simulink model "Orbits"  (R2017a)
settings: Solver=VariableStepAuto  StartTime=0.0  StopTime=5*orb_time  FixedStep=24*60*60  MaxStep=orb_time*5e-3  MinStep=5e-2  RelTol=1e-6  EnableMultiTasking=on
model workspace (MATLAB code in the model file):
  | Orbits_Setup
undefined symbols (not defined in the file or in its folder): C1, C2, dec_year, Earth, EIRSAT1, k01, k02, k03, orb_time, WGS84, X, Y, Z
libraries: sm_lib x18, nesl_utility x12, cstblocks x6, sharedtransform x3, aerolibtransform2 x1, aerolibgravity2 x1
Description:
  | Copyright 2008-2016 The MathWorks, Inc.
settings Model: Creator=MathWorks  LastModifiedBy=vicctorio
settings SolverCC: ZeroCrossControl=EnableAll
settings DataIOCC: SaveFormat=Array  OutputTimes=0  ReturnWorkspaceOutputsName=out2
settings OptimizationCC: LifeSpan=inf
settings DebuggingCC: UnderspecifiedInitializationDetection=Classic  MergeDetectMultiDrivingBlocksExec=none  SolverPrmCheckMsg=warning  SFUnexpectedBacktrackingDiag=warning  SFNoUnconditionalDefaultTransitionDiag=warning  SFExecutionAtInitializationDiag=none
settings HardwareCC: ProdBitPerPointer=32  ProdBitPerSizeT=32  ProdBitPerPtrDiffT=32  ProdLargestAtomicFloat=None  ProdIntDivRoundTo=Undefined  ProdEndianess=Unspecified  ProdWordSize=32  ProdHWDeviceType=32-bit Generic
settings ModelReferenceCC: PropagateSignalLabelsOutOfModel=off
settings GRTTargetCC: TargetLangStandard=C89/C90 (ANSI)  GeneratePreprocessorConditionals=Disable all
settings ConfigComp: CovMetricSettings=dw  CovHtmlReporting=on  CovSaveCumulativeToWorkspaceVar=on  CovSaveSingleToWorkspaceVar=on  CovExternalEMLEnable=off
settings SimscapeCC: SimscapeLogLimitData=off
settings ConfigurationSet: Description=SimMechanics 2G
settings ExplorerConfigSet: InternalSimMechanicsExplorerSettings="<ExplorerConfiguration><canonicalview>default</canonicalview><AnimationSetting><BasePlaybackSpeed>1e3</BasePlaybackSpeed><PlaybackSpeedFactor>1.0</PlaybackSpeedFactor></AnimationSetting><TilePanel><TileInfo><Tiles Columns=\"2\" Count=\"4\" Rows=\"2\"><Column Left=\"2\" Weight=\"0.5\"/><Column Left=\"393\" Weight=\"0.5\"/><Column Left=\"784\"/><Row Top=\"2\" Weight=\"0.5\"/><Row Top=\"345\" Weight=\"0.5\"/><Row Top=\"688\"/><Tile Height=\"1\" Width=\"1\" X=\"0\" Y=\"0\"/><Tile Height=\"1\" Width=\"1\" X=\"0\" Y=\"1\"/><Tile Height=\"1\" Width=\"1\" X=\"1\" Y=\"0\"/><Tile Height=\"1\" Width=\"1\" X=\"1\" Y=\"1\"/></Tiles></TileInfo><SceneInfo><SceneViewer><BGColor><R>0.901960790157318115</R><G>0.901960790157318115</G><B>0.901960790157318115</B></BGColor><Camera><DoPerspective>off</DoPerspective><Position><X>-203.545490264892578</X><Y>-167484806.482812434</Y><Z>-58.7216796875145519</Z></Position><Center><X>-203.545490264892578</X><Y>-83700.054443359375</Y><Z>-58.7216796875145519</Z></Center><Up><X>0</X><Y>-0</Y><Z>1</Z></Up><ViewLimDist>1</ViewLimDist><YLim>6562130</YLim><XLim>7505190.59880239516</XLim></Camera></SceneViewer><SceneViewer><BGColor><R>0.901960790157318115</R><G>0.901960790157318115</G><B>0.901960790157318115</B></BGColor><Camera><DoPerspective>off</DoPerspective><Position><X>-99808.0000004172325</X><Y>1.9073486328125e-06</Y><Z>11080569.0027875006</Z></Position><Center><X>-99808.0000004172325</X><Y>1.9073486328125e-06</Y><Z>1541215.53125</Z></Center><Up><X>0</X><Y>1</Y><Z>-0</Z></Up><ViewLimDist>1</ViewLimDist><YLim>7206500.06000000052</YLim><XLim>8242164.73928143829</XLim></Camera></SceneViewer><SceneViewer><BGColor><R>0.901960790157318115</R><G>0.901960790157318115</G><B>0.901960790157318115</B></BGColor><Camera><DoPerspective>off</DoPerspective><Position><X>1780793989.13458633</X><Y>-0.765625</Y><Z>0.0923618078231811523</Z></Position><Center><X>-1228213.1171875</X><Y>-0.765625</Y><Z>0.0923618078231811523</Z></Center><Up><X>-0</X><Y>0</Y><Z>1</Z></Up><ViewLimDist>1</ViewLimDist><YLim>6860208.48896073923</YLim><XLim>7846106.71491916943</XLim></Camera></SceneViewer><SceneViewer><BGColor><R>0.901960790157318115</R><G>0.901960790157318115</G><B>0.901960790157318115</B></BGColor><Camera><DoPerspective>off</DoPerspective><Position><X>1473413538.72739792</X><Y>-1473413538.82131076</Y><Z>1473411667.66141582</Z></Position><Center><X>-14.9597511113855024</X><Y>14.8658383234217677</Y><Z>-15.3674730430210413</Z></Center><Up><X>-0.408248290463863073</X><Y>0.408248290463863073</Y><Z>0.816496580927726145</Z></Up><ViewLimDist>1</ViewLimDist><YLim>10412227.7699999996</YLim><XLim>11908595.8327544909</XLim></Camera></SceneViewer></SceneInfo></TilePanel><MechEditorPanel><Cameras/><GfxPanelCameraMap/></MechEditorPanel></ExplorerConfiguration>"

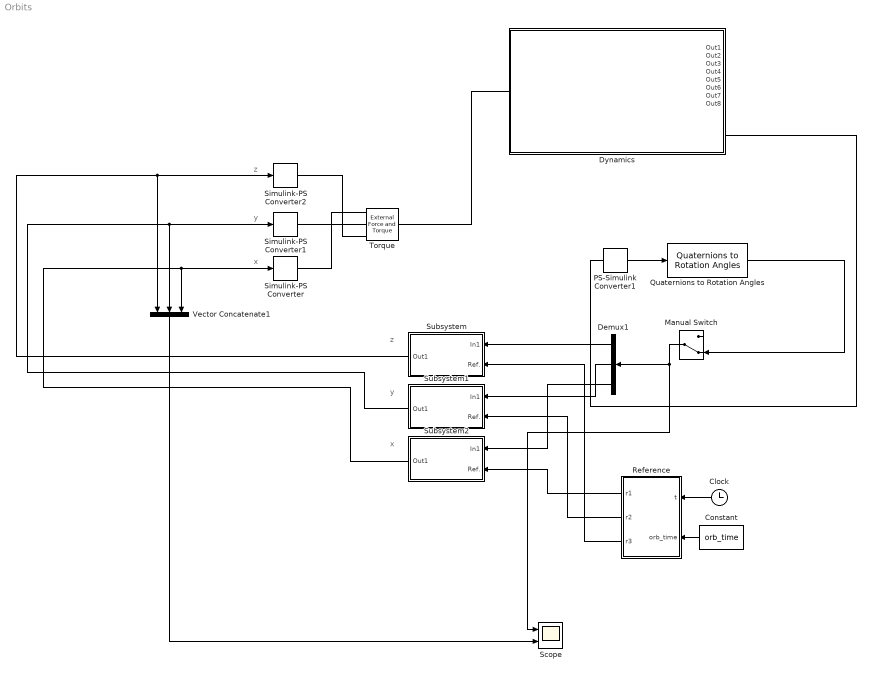
== system Orbits ==
  note: x
  note: y
  note: z
  note: x
  note: y
  note: z
  Clock : Clock
  Constant : Constant  Value=orb_time
  Demux1 : Demux  Outputs=3
  Dynamics : Subsystem
  Manual Switch : ManualSwitch  CurrentSetting=0
  PS-Simulink Converter1 : nesl_utility/PS-Simulink Converter  PhysicalDomain=network_engine_domain  SubClassName=ps_output  LeftPortType=input  RightPortType=output  PseudoPeriodic=off  Frequencies=[]  Unit=1  AffineConversion=off
  Quaternions to Rotation Angles : sharedtransform/Quaternions to Rotation Angles  rotationOrder=ZYX
  Reference : MATLAB Function  TreatAsAtomicUnit=on
  Scope : Scope  NumInputPorts=2
  Simulink-PS Converter : nesl_utility/Simulink-PS Converter  PhysicalDomain=network_engine_domain  SubClassName=ps_input  LeftPortType=input  RightPortType=output  PseudoPeriodic=off  Frequencies=[]  NoiseDistribution=none  NoiseParameters=[]  Unit=1  AffineConversion=off  FilteringAndDerivatives=zero  SimscapeFilterOrder=1  InputFilterTimeConstant=0.001  UdotUserProvided=1
  Simulink-PS Converter1 : nesl_utility/Simulink-PS Converter  PhysicalDomain=network_engine_domain  SubClassName=ps_input  LeftPortType=input  RightPortType=output  PseudoPeriodic=off  Frequencies=[]  NoiseDistribution=none  NoiseParameters=[]  Unit=1  AffineConversion=off  FilteringAndDerivatives=zero  SimscapeFilterOrder=1  InputFilterTimeConstant=0.001  UdotUserProvided=1
  Simulink-PS Converter2 : nesl_utility/Simulink-PS Converter  PhysicalDomain=network_engine_domain  SubClassName=ps_input  LeftPortType=input  RightPortType=output  PseudoPeriodic=off  Frequencies=[]  NoiseDistribution=none  NoiseParameters=[]  Unit=1  AffineConversion=off  FilteringAndDerivatives=zero  SimscapeFilterOrder=1  InputFilterTimeConstant=0.001  UdotUserProvided=1
  Subsystem : Subsystem
  Subsystem1 : Subsystem
  Subsystem2 : Subsystem
  Torque : sm_lib/Forces and Torques/External Force and Torque  ForceResolutionFrame=AttachedFrame  EnableForceX=off  EnableForceY=off  EnableForceZ=off  EnableForce=off  TorqueResolutionFrame=AttachedFrame  EnableTorqueX=on  EnableTorqueY=on  EnableTorqueZ=on  EnableTorque=off
  Vector Concatenate1 : Concatenate  NumInputs=3
  wires:
  PS-Simulink Converter1/1 -> Quaternions to Rotation Angles/1
  Demux1/2 -> Subsystem1/1(In1)
  Demux1/1 -> Subsystem/1(In1)
  Demux1/3 -> Subsystem2/1(In1)
  Quaternions to Rotation Angles/1 -> Manual Switch/2
  Vector Concatenate1/1 -> Scope/2
  Manual Switch/1 -> Scope/1, Demux1/1
  Clock/1 -> Reference/1(t)
  Constant/1 -> Reference/2(orb_time)
  Reference/2(r2) -> Subsystem1/2(Ref.)
  Reference/1(r1) -> Subsystem2/2(Ref.)
  Reference/3(r3) -> Subsystem/2(Ref.)
  Subsystem/1(Out1) -> Simulink-PS Converter2/1, Vector Concatenate1/1
  Subsystem1/1(Out1) -> Simulink-PS Converter1/1, Vector Concatenate1/2
  Subsystem2/1(Out1) -> Simulink-PS Converter/1, Vector Concatenate1/3
  connections:
  Simulink-PS Converter1/RConn1 -- Torque/LConn2
  Simulink-PS Converter/RConn1 -- Torque/LConn1
  Simulink-PS Converter2/RConn1 -- Torque/LConn3
  Torque/RConn1 -- Dynamics/LConn1
  Dynamics/RConn4 -- PS-Simulink Converter1/LConn1

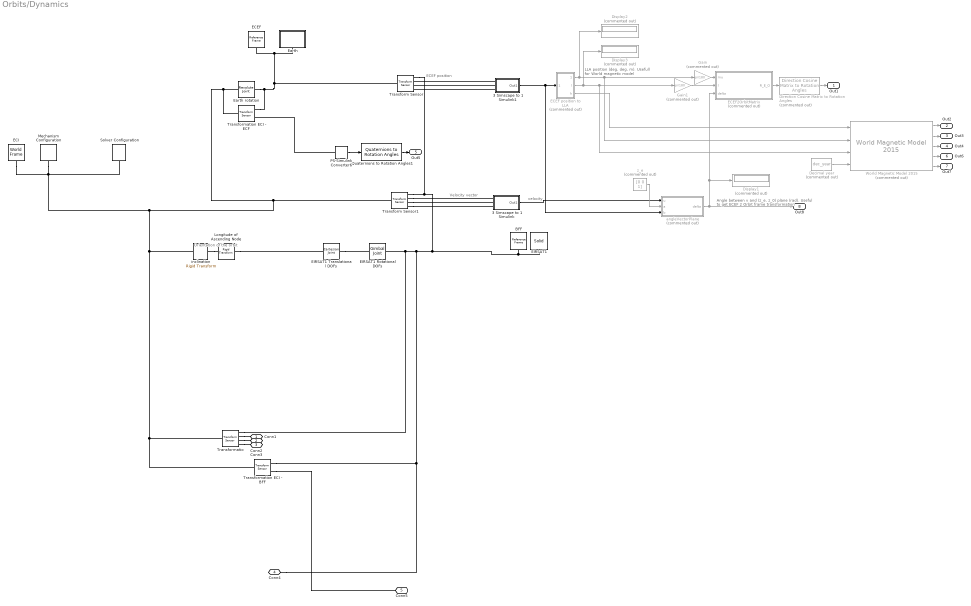
== system Orbits/Dynamics ==
  note: LLA position (deg, deg, m).
      | Usefull for World magnetic model
  note: Angle between v and (z_e, z_0) plane (rad).
      | Useful to get ECEF 2 Orbit frame transformation
  note: velocity
  note: Velocity vector
  note: ECEF position
  note: Orientation of the orbit
  " Earth rotation" : sm_lib/Joints/Revolute Joint  SenseConstraintForce=off  SenseConstraintForceX=off  SenseConstraintForceY=off  SenseConstraintForceZ=off  SenseConstraintTorque=off  SenseConstraintTorqueX=off  SenseConstraintTorqueY=off  SenseConstraintTorqueZ=off  SenseTotalForce=off  SenseTotalForceX=off  SenseTotalForceY=off  SenseTotalForceZ=off  SenseTotalTorque=off  SenseTotalTorqueX=off  SenseTotalTorqueY=off  SenseTotalTorqueZ=off  CompositeWrenchDir=FollowerOnBase  CompositeWrenchFrame=BaseFrame  EquilibriumPosition=0  EquilibriumPositionUnits=deg  SpringStiffness=0  SpringStiffnessUnits=N*m/deg  DampingCoefficient=0  DampingCoefficientUnits=N*m/(deg/s)  TorqueActuationMode=NoTorque  MotionActuationMode=ComputedMotion  SensePosition=off  SenseVelocity=off  SenseAcceleration=off  SenseTorqueForce=off  PositionTargetSpecify=off  PositionTargetPriority=High  PositionTargetValue=0  PositionTargetValueUnits=deg  VelocityTargetSpecify=on  VelocityTargetPriority=High  VelocityTargetValue=Earth.w  VelocityTargetValueUnits=deg/s
  3 Simscape to 1 Simulink : Subsystem
  3 Simscape to 1 Simulink1 : Subsystem
  BFF : sm_lib/Frames and Transforms/Reference Frame
  Decimal year : Constant  Commented=on  Value=dec_year
  Direction Cosine Matrix to Rotation Angles : sharedtransform/Direction Cosine Matrix to Rotation Angles  Commented=on  rotationOrder=ZYX  lim=Default
  Display1 : Display  Commented=on
  Display2 : Display  Commented=on
  Display3 : Display  Commented=on
  "ECEF " : sm_lib/Frames and Transforms/Reference Frame
  ECEF position to LLA : Subsystem  Commented=on
  ECEF2OrbitMatrix : MATLAB Function  Commented=on  TreatAsAtomicUnit=on
  ECI : sm_lib/Frames and Transforms/World Frame
  EIRSAT1 : sm_lib/Body Elements/Solid  InertiaType=Custom  Mass=EIRSAT1.M  MassUnits=kg  CenterOfMass=EIRSAT1.COM  CenterOfMassUnits=m  MomentsOfInertia=EIRSAT1.MomI  MomentsOfInertiaUnits=kg*m^2  ProductsOfInertia=EIRSAT1.ProdI  ProductsOfInertiaUnits=kg*m^2  DensityBased=off  Density=1000  DensityUnits=kg/(m^3)  DoExposeReferenceFrame=on  SerializedFrames=<Frames/>  GraphicType=FromGeometry  MarkerShape=Sphere  MarkerSize=10  MarkerSizeUnits=m  GraphicVisPropType=SimpleVisualProperties  GraphicDiffuseColor=EIRSAT1.RGB  GraphicSpecularColor=[0.5 0.5 0.5 1.0]  GraphicAmbientColor=[0.15 0.15 0.15 1.0]  GraphicEmissiveColor=[0.0 0.0 0.0 1.0]  GraphicShininess=75  GraphicOpacity=1.0  GeometryShape=Brick  RectangleSize=[1 1]  RectangleSizeUnits=m  BrickDimensions=[1 1 2] * EIRSAT1.R  BrickDimensionUnits=m  CylinderRadius=1  CylinderRadiusUnits=m  CylinderLength=1  CylinderLengthUnits=m  SphereRadius=EIRSAT1.R  SphereRadiusUnits=m  EllipsoidRadii=[1 1 1]  EllipsoidRadiiUnits=m  ExtrusionCrossSection=[1 1; -1 1; -1 -1; 1 -1]  ExtrusionCrossSectionUnits=m  ExtrusionLength=1  ExtrusionLengthUnits=m  PolygonNumSides=3  PolygonOuterRadius=1  PolygonOuterRadiusUnits=m  ExtGeomFileType=STL  ExtGeomFileUnits=m  RevolutionCrossSection=[1 1; 1 -1; 2 -1; 2 1]  RevolutionCrossSectionUnits=m  RevolutionExtent=Full  RevolutionAngle=180  RevolutionAngleUnits=deg
  EIRSAT1 Rotational DOFs : sm_lib/Joints/Gimbal Joint  SenseConstraintForce=off  SenseConstraintForceX=off  SenseConstraintForceY=off  SenseConstraintForceZ=off  SenseConstraintTorque=off  SenseConstraintTorqueX=off  SenseConstraintTorqueY=off  SenseConstraintTorqueZ=off  SenseTotalForce=off  SenseTotalForceX=off  SenseTotalForceY=off  SenseTotalForceZ=off  SenseTotalTorque=off  SenseTotalTorqueX=off  SenseTotalTorqueY=off  SenseTotalTorqueZ=off  CompositeWrenchDir=FollowerOnBase  CompositeWrenchFrame=BaseFrame  RxEquilibriumPosition=0  RxEquilibriumPositionUnits=deg  RxSpringStiffness=0  RxSpringStiffnessUnits=N*m/deg  RxDampingCoefficient=0  RxDampingCoefficientUnits=N*m/(deg/s)  RxTorqueActuationMode=NoTorque  RxMotionActuationMode=ComputedMotion  RxSensePosition=off  RxSenseVelocity=off  RxSenseAcceleration=off  RxSenseTorqueForce=off  RxPositionTargetSpecify=off  RxPositionTargetPriority=High  RxPositionTargetValue=0  RxPositionTargetValueUnits=deg  RxVelocityTargetSpecify=off  RxVelocityTargetPriority=High  RxVelocityTargetValue=0.2  RxVelocityTargetValueUnits=rad/s  RyEquilibriumPosition=0  RyEquilibriumPositionUnits=deg  RySpringStiffness=0  RySpringStiffnessUnits=N*m/deg  RyDampingCoefficient=0  RyDampingCoefficientUnits=N*m/(deg/s)  RyTorqueActuationMode=NoTorque  RyMotionActuationMode=ComputedMotion  RySensePosition=off  RySenseVelocity=off  RySenseAcceleration=off  RySenseTorqueForce=off  RyPositionTargetSpecify=off  RyPositionTargetPriority=High  RyPositionTargetValue=0  RyPositionTargetValueUnits=deg  RyVelocityTargetSpecify=off  RyVelocityTargetPriority=High  RyVelocityTargetValue=0.1  RyVelocityTargetValueUnits=deg/s  RzEquilibriumPosition=0  RzEquilibriumPositionUnits=deg  RzSpringStiffness=0  RzSpringStiffnessUnits=N*m/deg  RzDampingCoefficient=0  RzDampingCoefficientUnits=N*m/(deg/s)  RzTorqueActuationMode=NoTorque  RzMotionActuationMode=ComputedMotion  RzSensePosition=off  RzSenseVelocity=off  RzSenseAcceleration=off  RzSenseTorqueForce=off  RzPositionTargetSpecify=off  RzPositionTargetPriority=High  RzPositionTargetValue=0  RzPositionTargetValueUnits=deg  RzVelocityTargetSpecify=off  RzVelocityTargetPriority=High  RzVelocityTargetValue=0.1  RzVelocityTargetValueUnits=deg/s
      settings: SourceProductName=Simscape Multibody
  EIRSAT1 Translational DOFs : sm_lib/Joints/Cartesian Joint  SenseConstraintForce=off  SenseConstraintForceX=off  SenseConstraintForceY=off  SenseConstraintForceZ=off  SenseConstraintTorque=off  SenseConstraintTorqueX=off  SenseConstraintTorqueY=off  SenseConstraintTorqueZ=off  SenseTotalForce=off  SenseTotalForceX=off  SenseTotalForceY=off  SenseTotalForceZ=off  SenseTotalTorque=off  SenseTotalTorqueX=off  SenseTotalTorqueY=off  SenseTotalTorqueZ=off  CompositeWrenchDir=FollowerOnBase  CompositeWrenchFrame=BaseFrame  PxEquilibriumPosition=0  PxEquilibriumPositionUnits=m  PxSpringStiffness=0  PxSpringStiffnessUnits=N/m  PxDampingCoefficient=0  PxDampingCoefficientUnits=N/(m/s)  PxTorqueActuationMode=NoTorque  PxMotionActuationMode=ComputedMotion  PxSensePosition=off  PxSenseVelocity=off  PxSenseAcceleration=off  PxSenseTorqueForce=off  PxPositionTargetSpecify=on  PxPositionTargetPriority=High  PxPositionTargetValue=EIRSAT1.Px  PxPositionTargetValueUnits=m  PxVelocityTargetSpecify=on  PxVelocityTargetPriority=High  PxVelocityTargetValue=EIRSAT1.Vx  PxVelocityTargetValueUnits=m/s  PyEquilibriumPosition=0  PyEquilibriumPositionUnits=m  PySpringStiffness=0  PySpringStiffnessUnits=N/m  PyDampingCoefficient=0  PyDampingCoefficientUnits=N/(m/s)  PyTorqueActuationMode=NoTorque  PyMotionActuationMode=ComputedMotion  PySensePosition=off  PySenseVelocity=off  PySenseAcceleration=off  PySenseTorqueForce=off  PyPositionTargetSpecify=on  PyPositionTargetPriority=High  PyPositionTargetValue=EIRSAT1.Py  PyPositionTargetValueUnits=m  PyVelocityTargetSpecify=on  PyVelocityTargetPriority=High  PyVelocityTargetValue=EIRSAT1.Vy  PyVelocityTargetValueUnits=m/s  PzEquilibriumPosition=0  PzEquilibriumPositionUnits=m  PzSpringStiffness=0  PzSpringStiffnessUnits=N/m  PzDampingCoefficient=0  PzDampingCoefficientUnits=N/(m/s)  PzTorqueActuationMode=NoTorque  PzMotionActuationMode=ComputedMotion  PzSensePosition=off  PzSenseVelocity=off  PzSenseAcceleration=off  PzSenseTorqueForce=off  PzPositionTargetSpecify=off  PzPositionTargetPriority=High  PzPositionTargetValue=0  PzPositionTargetValueUnits=m  PzVelocityTargetSpecify=off  PzVelocityTargetPriority=High  PzVelocityTargetValue=0  PzVelocityTargetValueUnits=m/s
  Earth : Subsystem
  Gain : Gain  Commented=on  Gain=pi/180
  Gain1 : Gain  Commented=on  Gain=pi/180
  Longitude of Ascending Node : sm_lib/Frames and Transforms/Rigid Transform  TranslationMethod=None  TranslationStandardOffset=0  TranslationLengthUnit=m  TranslationStandardAxis=+Z  TranslationCartesianOffset=[0 0 0]  TranslationROffset=0  TranslationROffsetUnits=m  TranslationZOffset=0  TranslationZOffsetUnits=m  TranslationThetaOffset=0  TranslationThetaOffsetUnits=deg  RotationMethod=StandardAxis  RotationAngleUnits=deg  RotationStandardAxis=+Z  RotationAngle=48.33  RotationArbitraryAxis=[0 0 1]  FollAlignAxisA=+X  BaseAlignAxisA=+Y  FollAlignAxisB=+Y  BaseAlignAxisB=+Z  RotationSequenceAxes=FollowerAxes  RotationSequence=XYX  RotationSequenceAngles=[0 0 0]  RotationSequenceAnglesUnits=deg  RotationMatrix=[1 0 0; 0 1 0; 0 0 1]
  Mechanism Configuration : sm_lib/Utilities/Mechanism Configuration  UniformGravity=None  GravityVector=[0 0 -9.80665]  GravityUnits=m/s^2  LinearizationDelta=0.001
  PS-Simulink Converter6 : nesl_utility/PS-Simulink Converter  PhysicalDomain=network_engine_domain  SubClassName=ps_output  LeftPortType=input  RightPortType=output  PseudoPeriodic=off  Frequencies=[]  Unit=1  AffineConversion=off
  Quaternions to Rotation Angles1 : sharedtransform/Quaternions to Rotation Angles  rotationOrder=ZYX
  Solver Configuration : nesl_utility/Solver Configuration  PhysicalDomain=network_engine_domain  SubClassName=solver  LeftPortType=input  RightPortType=generic  Accelerate=off  Tones=[]  Harmonics=[]  SimulateNoise=off  Profile=off  UseLocalSampling=off  EnableSwitchedLinearOptims=on  FrequencyDomain=off  UseCCode=off  RelTol=0.001  AbsTol=1e-06  MinStep=1e-09  ToWorkspace=off  RevertToSquareIcSolve=off  NumHomotopyIterations=100  PhasorMode=off  PhasorModeNumHarmonics=1  OverrideAbsTol=off  DoDC=off  ResidualTolerance=1e-09  UseLocalSolver=off  LocalSolverChoice=NE_BACKWARD_EULER_ADVANCER  LocalSolverSampleTime=0.001  DoFixedCost=off  MaxNonlinIter=3  MaxModeIter=2  LinearAlgebra=Sparse  DelaysMemoryBudget=1024  AutomaticFiltering=on  FilteringTimeConstant=0.001
  Transform Sensor : sm_lib/Frames and Transforms/Transform Sensor  MeasurementFrame=World  SenseAngle=off  SenseAxis=off  SenseAngle1=off  SenseAngle2=off  SenseAngle3=off  SenseQ=off  SenseR=off  SenseOmegaX=off  SenseOmegaY=off  SenseOmegaZ=off  SenseOmega1=off  SenseOmega2=off  SenseOmega3=off  SenseQDot=off  SenseRDot=off  SenseAlphaX=off  SenseAlphaY=off  SenseAlphaZ=off  SenseAlpha1=off  SenseAlpha2=off  SenseAlpha3=off  SenseQDDot=off  SenseRDDot=off  SenseX=on  SenseY=on  SenseZ=on  SenseRad=off  SenseAzim=off  SenseDist=off  SenseInc=off  SenseXDot=off  SenseYDot=off  SenseZDot=off  SenseRadDot=off  SenseAzimDot=off  SenseDistDot=off  SenseIncDot=off  SenseXDDot=off  SenseYDDot=off  SenseZDDot=off  SenseRadDDot=off  SenseAzimDDot=off  SenseDistDDot=off  SenseIncDDot=off
  Transform Sensor1 : sm_lib/Frames and Transforms/Transform Sensor  MeasurementFrame=World  SenseAngle=off  SenseAxis=off  SenseAngle1=off  SenseAngle2=off  SenseAngle3=off  SenseQ=off  SenseR=off  SenseOmegaX=off  SenseOmegaY=off  SenseOmegaZ=off  SenseOmega1=off  SenseOmega2=off  SenseOmega3=off  SenseQDot=off  SenseRDot=off  SenseAlphaX=off  SenseAlphaY=off  SenseAlphaZ=off  SenseAlpha1=off  SenseAlpha2=off  SenseAlpha3=off  SenseQDDot=off  SenseRDDot=off  SenseX=off  SenseY=off  SenseZ=off  SenseRad=off  SenseAzim=off  SenseDist=off  SenseInc=off  SenseXDot=on  SenseYDot=on  SenseZDot=on  SenseRadDot=off  SenseAzimDot=off  SenseDistDot=off  SenseIncDot=off  SenseXDDot=off  SenseYDDot=off  SenseZDDot=off  SenseRadDDot=off  SenseAzimDDot=off  SenseDistDDot=off  SenseIncDDot=off
  Transformatio : sm_lib/Frames and Transforms/Transform Sensor  MeasurementFrame=World  SenseAngle=off  SenseAxis=off  SenseAngle1=off  SenseAngle2=off  SenseAngle3=off  SenseQ=off  SenseR=off  SenseOmegaX=off  SenseOmegaY=off  SenseOmegaZ=off  SenseOmega1=off  SenseOmega2=off  SenseOmega3=off  SenseQDot=off  SenseRDot=off  SenseAlphaX=off  SenseAlphaY=off  SenseAlphaZ=off  SenseAlpha1=off  SenseAlpha2=off  SenseAlpha3=off  SenseQDDot=off  SenseRDDot=off  SenseX=on  SenseY=on  SenseZ=on  SenseRad=off  SenseAzim=off  SenseDist=off  SenseInc=off  SenseXDot=off  SenseYDot=off  SenseZDot=off  SenseRadDot=off  SenseAzimDot=off  SenseDistDot=off  SenseIncDot=off  SenseXDDot=off  SenseYDDot=off  SenseZDDot=off  SenseRadDDot=off  SenseAzimDDot=off  SenseDistDDot=off  SenseIncDDot=off
  Transformation ECI - BFF : sm_lib/Frames and Transforms/Transform Sensor  MeasurementFrame=World  SenseAngle=off  SenseAxis=off  SenseAngle1=off  SenseAngle2=off  SenseAngle3=off  SenseQ=on  SenseR=off  SenseOmegaX=off  SenseOmegaY=off  SenseOmegaZ=off  SenseOmega1=off  SenseOmega2=off  SenseOmega3=off  SenseQDot=off  SenseRDot=off  SenseAlphaX=off  SenseAlphaY=off  SenseAlphaZ=off  SenseAlpha1=off  SenseAlpha2=off  SenseAlpha3=off  SenseQDDot=off  SenseRDDot=off  SenseX=off  SenseY=off  SenseZ=off  SenseRad=off  SenseAzim=off  SenseDist=off  SenseInc=off  SenseXDot=off  SenseYDot=off  SenseZDot=off  SenseRadDot=off  SenseAzimDot=off  SenseDistDot=off  SenseIncDot=off  SenseXDDot=off  SenseYDDot=off  SenseZDDot=off  SenseRadDDot=off  SenseAzimDDot=off  SenseDistDDot=off  SenseIncDDot=off
  Transformation ECI - ECF : sm_lib/Frames and Transforms/Transform Sensor  MeasurementFrame=World  SenseAngle=off  SenseAxis=off  SenseAngle1=off  SenseAngle2=off  SenseAngle3=off  SenseQ=on  SenseR=off  SenseOmegaX=off  SenseOmegaY=off  SenseOmegaZ=off  SenseOmega1=off  SenseOmega2=off  SenseOmega3=off  SenseQDot=off  SenseRDot=off  SenseAlphaX=off  SenseAlphaY=off  SenseAlphaZ=off  SenseAlpha1=off  SenseAlpha2=off  SenseAlpha3=off  SenseQDDot=off  SenseRDDot=off  SenseX=off  SenseY=off  SenseZ=off  SenseRad=off  SenseAzim=off  SenseDist=off  SenseInc=off  SenseXDot=off  SenseYDot=off  SenseZDot=off  SenseRadDot=off  SenseAzimDot=off  SenseDistDot=off  SenseIncDot=off  SenseXDDot=off  SenseYDDot=off  SenseZDDot=off  SenseRadDDot=off  SenseAzimDDot=off  SenseDistDDot=off  SenseIncDDot=off
  World Magnetic Model 2015 : aerolibgravity2/World Magnetic Model 2015  Commented=on  units=Metric (MKS)  time_in=on  month=January  day=1  year=2015  action=Error  h_out=on  dec_out=on  inc_out=on  ti_out=on
      settings: SourceProductName=Aerospace Blockset  SourceProductBaseCode=AE
  angleVectorPlane : MATLAB Function  Commented=on  TreatAsAtomicUnit=on
  inclination : sm_lib/Frames and Transforms/Rigid Transform  TranslationMethod=None  TranslationStandardOffset=0  TranslationLengthUnit=m  TranslationStandardAxis=+Z  TranslationCartesianOffset=[0 0 0]  TranslationROffset=0  TranslationROffsetUnits=m  TranslationZOffset=0  TranslationZOffsetUnits=m  TranslationThetaOffset=0  TranslationThetaOffsetUnits=deg  RotationMethod=StandardAxis  RotationAngleUnits=deg  RotationStandardAxis=+X  RotationAngle=20  RotationArbitraryAxis=[0 0 1]  FollAlignAxisA=+X  BaseAlignAxisA=+Y  FollAlignAxisB=+Y  BaseAlignAxisB=+Z  RotationSequenceAxes=FollowerAxes  RotationSequence=XYX  RotationSequenceAngles=[0 0 0]  RotationSequenceAnglesUnits=deg  RotationMatrix=[1 0 0; 0 1 0; 0 0 1]
  z_e : Constant  Commented=on  Value=[0 0 1]
  Conn1 : PMIOPort  Port=1  Side=Right
  Conn2 : PMIOPort  Port=2  Side=Right
  Conn3 : PMIOPort  Port=3  Side=Right
  Conn4 : PMIOPort  Port=4  Side=Left
  Conn5 : PMIOPort  Port=5  Side=Right
  Out1 : Outport
  Out2 : Outport  Port=2
  Out3 : Outport  Port=3
  Out4 : Outport  Port=4
  Out5 : Outport  Port=5
  Out6 : Outport  Port=6
  Out7 : Outport  Port=7
  Out8 : Outport  Port=8
  wires:
  PS-Simulink Converter6/1 -> Quaternions to Rotation Angles1/1
  3 Simscape to 1 Simulink/1(Out1) -> angleVectorPlane/1(u)
  ECEF position to LLA/2(l) -> Display3/1, World Magnetic Model 2015/3, Gain1/1
  3 Simscape to 1 Simulink1/1(Out1) -> angleVectorPlane/3(b), ECEF position to LLA/1(In1)
  Gain1/1 -> ECEF2OrbitMatrix/2(l)
  z_e/1 -> angleVectorPlane/2(a)
  angleVectorPlane/1(delta) -> Out8/1, ECEF2OrbitMatrix/3(delta), Display1/1
  Decimal year/1 -> World Magnetic Model 2015/4
  ECEF position to LLA/3(h) -> World Magnetic Model 2015/1
  ECEF2OrbitMatrix/1(R_E_O) -> Direction Cosine Matrix to Rotation Angles/1
  ECEF position to LLA/1(mu) -> Gain/1, World Magnetic Model 2015/2, Display2/1
  Gain/1 -> ECEF2OrbitMatrix/1(mu)
  World Magnetic Model 2015/3 -> Out4/1
  Quaternions to Rotation Angles1/1 -> Out5/1
  World Magnetic Model 2015/1 -> Out2/1
  World Magnetic Model 2015/4 -> Out6/1
  World Magnetic Model 2015/5 -> Out7/1
  Direction Cosine Matrix to Rotation Angles/1 -> Out1/1
  World Magnetic Model 2015/2 -> Out3/1
  connections:
  Transformation ECI - BFF/RConn2 -- Conn5/RConn1
  inclination/RConn1 -- Longitude of Ascending Node/LConn1
  inclination/LConn1 -- Transformatio/LConn1 -- Transformation ECI - BFF/LConn1 -- " Earth rotation"/LConn1 -- Transformation ECI - ECF/LConn1 -- Transform Sensor1/LConn1 -- Solver Configuration/RConn1 -- ECI/RConn1 -- Mechanism Configuration/RConn1
  Transformation ECI - BFF/RConn1 -- Conn4/RConn1 -- EIRSAT1/RConn1 -- BFF/RConn1 -- Transform Sensor/RConn1 -- Transform Sensor1/RConn1 -- Transformatio/RConn1 -- EIRSAT1 Rotational DOFs/RConn1
  Longitude of Ascending Node/RConn1 -- EIRSAT1 Translational DOFs/LConn1
  PS-Simulink Converter6/LConn1 -- Transformation ECI - ECF/RConn2
  " Earth rotation"/RConn1 -- Transform Sensor/LConn1 -- Earth/LConn1 -- "ECEF "/RConn1 -- Transformation ECI - ECF/RConn1
  Transform Sensor1/RConn4 -- 3 Simscape to 1 Simulink/LConn3
  Transform Sensor1/RConn2 -- 3 Simscape to 1 Simulink/LConn1
  EIRSAT1 Translational DOFs/RConn1 -- EIRSAT1 Rotational DOFs/LConn1
  Transform Sensor1/RConn3 -- 3 Simscape to 1 Simulink/LConn2
  3 Simscape to 1 Simulink1/LConn3 -- Transform Sensor/RConn4
  3 Simscape to 1 Simulink1/LConn1 -- Transform Sensor/RConn2
  3 Simscape to 1 Simulink1/LConn2 -- Transform Sensor/RConn3
  Transformatio/RConn2 -- Conn1/RConn1
  Transformatio/RConn3 -- Conn2/RConn1
  Transformatio/RConn4 -- Conn3/RConn1

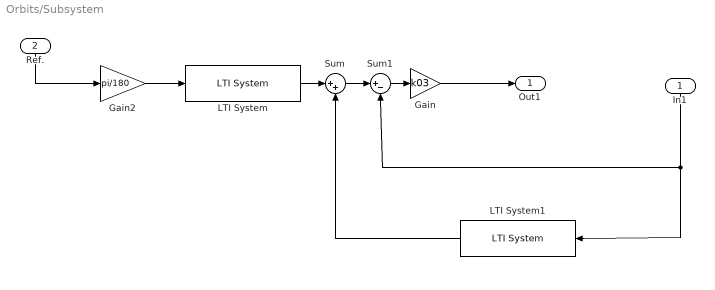
== system Orbits/Subsystem ==
  In1 : Inport
  Ref. : Inport  Port=2
  Gain : Gain  Gain=k03
  Gain2 : Gain  Gain=pi/180
  LTI System : cstblocks/LTI System  sys=C1(3)  IC=[]
  LTI System1 : cstblocks/LTI System  sys=C2(3)  IC=[]
  Sum : Sum  Inputs=|++
  Sum1 : Sum  Inputs=|+-
  Out1 : Outport
  wires:
  Sum1/1 -> Gain/1
  LTI System/1 -> Sum/1
  LTI System1/1 -> Sum/2
  Sum/1 -> Sum1/1
  In1/1 -> LTI System1/1, Sum1/2
  Gain2/1 -> LTI System/1
  Gain/1 -> Out1/1
  Ref./1 -> Gain2/1

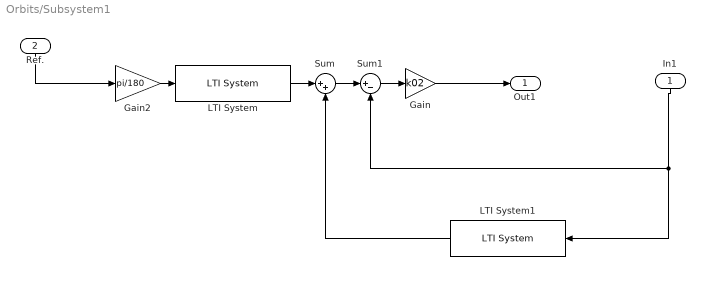
== system Orbits/Subsystem1 ==
  In1 : Inport
  Ref. : Inport  Port=2
  Gain : Gain  Gain=k02
  Gain2 : Gain  Gain=pi/180
  LTI System : cstblocks/LTI System  sys=C1(2)  IC=[]
  LTI System1 : cstblocks/LTI System  sys=C2(2)  IC=[]
  Sum : Sum  Inputs=|++
  Sum1 : Sum  Inputs=|+-
  Out1 : Outport
  wires:
  Sum1/1 -> Gain/1
  LTI System/1 -> Sum/1
  LTI System1/1 -> Sum/2
  Sum/1 -> Sum1/1
  In1/1 -> LTI System1/1, Sum1/2
  Gain2/1 -> LTI System/1
  Gain/1 -> Out1/1
  Ref./1 -> Gain2/1

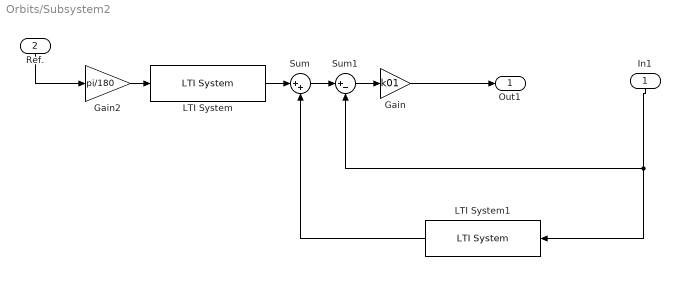
== system Orbits/Subsystem2 ==
  In1 : Inport
  Ref. : Inport  Port=2
  Gain : Gain  Gain=k01
  Gain2 : Gain  Gain=pi/180
  LTI System : cstblocks/LTI System  sys=C1(1)  IC=[]
  LTI System1 : cstblocks/LTI System  sys=C2(1)  IC=[]
  Sum : Sum  Inputs=|++
  Sum1 : Sum  Inputs=|+-
  Out1 : Outport
  wires:
  Sum1/1 -> Gain/1
  LTI System/1 -> Sum/1
  LTI System1/1 -> Sum/2
  Sum/1 -> Sum1/1
  In1/1 -> LTI System1/1, Sum1/2
  Gain/1 -> Out1/1
  Gain2/1 -> LTI System/1
  Ref./1 -> Gain2/1

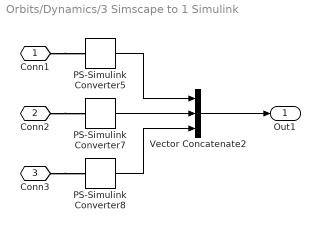
== system Orbits/Dynamics/3 Simscape to 1 Simulink ==
  PS-Simulink Converter5 : nesl_utility/PS-Simulink Converter  PhysicalDomain=network_engine_domain  SubClassName=ps_output  LeftPortType=input  RightPortType=output  PseudoPeriodic=off  Frequencies=[]  Unit=1  AffineConversion=off
  PS-Simulink Converter7 : nesl_utility/PS-Simulink Converter  PhysicalDomain=network_engine_domain  SubClassName=ps_output  LeftPortType=input  RightPortType=output  PseudoPeriodic=off  Frequencies=[]  Unit=1  AffineConversion=off
  PS-Simulink Converter8 : nesl_utility/PS-Simulink Converter  PhysicalDomain=network_engine_domain  SubClassName=ps_output  LeftPortType=input  RightPortType=output  PseudoPeriodic=off  Frequencies=[]  Unit=1  AffineConversion=off
  Vector Concatenate2 : Concatenate  NumInputs=3
  Conn1 : PMIOPort  Port=1  Side=Left
  Conn2 : PMIOPort  Port=2  Side=Left
  Conn3 : PMIOPort  Port=3  Side=Left
  Out1 : Outport
  wires:
  PS-Simulink Converter5/1 -> Vector Concatenate2/1
  PS-Simulink Converter7/1 -> Vector Concatenate2/2
  PS-Simulink Converter8/1 -> Vector Concatenate2/3
  Vector Concatenate2/1 -> Out1/1
  connections:
  Conn3/RConn1 -- PS-Simulink Converter8/LConn1
  Conn2/RConn1 -- PS-Simulink Converter7/LConn1
  Conn1/RConn1 -- PS-Simulink Converter5/LConn1

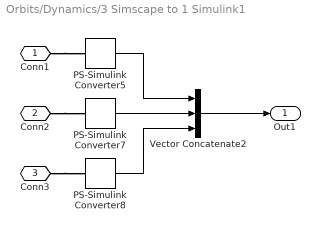
== system Orbits/Dynamics/3 Simscape to 1 Simulink1 ==
  PS-Simulink Converter5 : nesl_utility/PS-Simulink Converter  PhysicalDomain=network_engine_domain  SubClassName=ps_output  LeftPortType=input  RightPortType=output  PseudoPeriodic=off  Frequencies=[]  Unit=1  AffineConversion=off
  PS-Simulink Converter7 : nesl_utility/PS-Simulink Converter  PhysicalDomain=network_engine_domain  SubClassName=ps_output  LeftPortType=input  RightPortType=output  PseudoPeriodic=off  Frequencies=[]  Unit=1  AffineConversion=off
  PS-Simulink Converter8 : nesl_utility/PS-Simulink Converter  PhysicalDomain=network_engine_domain  SubClassName=ps_output  LeftPortType=input  RightPortType=output  PseudoPeriodic=off  Frequencies=[]  Unit=1  AffineConversion=off
  Vector Concatenate2 : Concatenate  NumInputs=3
  Conn1 : PMIOPort  Port=1  Side=Left
  Conn2 : PMIOPort  Port=2  Side=Left
  Conn3 : PMIOPort  Port=3  Side=Left
  Out1 : Outport
  wires:
  PS-Simulink Converter5/1 -> Vector Concatenate2/1
  PS-Simulink Converter7/1 -> Vector Concatenate2/2
  PS-Simulink Converter8/1 -> Vector Concatenate2/3
  Vector Concatenate2/1 -> Out1/1
  connections:
  Conn3/RConn1 -- PS-Simulink Converter8/LConn1
  Conn2/RConn1 -- PS-Simulink Converter7/LConn1
  Conn1/RConn1 -- PS-Simulink Converter5/LConn1

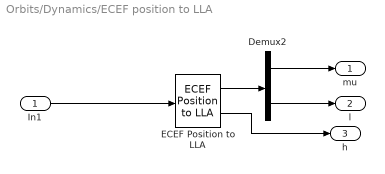
== system Orbits/Dynamics/ECEF position to LLA ==
  In1 : Inport
  Demux2 : Demux  Outputs=2
  ECEF Position to LLA : aerolibtransform2/ECEF Position to LLA  units=Metric (MKS)  ptype=Earth (WGS84)  F=1/298.257223563  R=6378137
      settings: SourceProductName=Aerospace Blockset  SourceProductBaseCode=AE
  mu : Outport
  l : Outport  Port=2
  h : Outport  Port=3
  wires:
  Demux2/2 -> l/1
  Demux2/1 -> mu/1
  ECEF Position to LLA/2 -> h/1
  In1/1 -> ECEF Position to LLA/1
  ECEF Position to LLA/1 -> Demux2/1

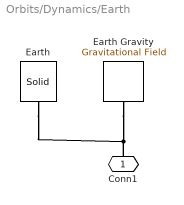
== system Orbits/Dynamics/Earth ==
  Earth : sm_lib/Body Elements/Solid  InertiaType=CalculateFromGeometry  Mass=Earth.M  MassUnits=kg  CenterOfMass=[0 0 0]  CenterOfMassUnits=m  MomentsOfInertia=[1 1 1]  MomentsOfInertiaUnits=kg*m^2  ProductsOfInertia=[0 0 0]  ProductsOfInertiaUnits=kg*m^2  DensityBased=off  Density=1000  DensityUnits=kg/(m^3)  DoExposeReferenceFrame=on  SerializedFrames=<Frames/>  GraphicType=FromGeometry  MarkerShape=Sphere  MarkerSize=10  MarkerSizeUnits=m  GraphicVisPropType=SimpleVisualProperties  GraphicDiffuseColor=Earth.RGB  GraphicSpecularColor=[0.5 0.5 0.5 1.0]  GraphicAmbientColor=[0.15 0.15 0.15 1.0]  GraphicEmissiveColor=[0.0 0.0 0.0 1.0]  GraphicShininess=75  GraphicOpacity=1.0  GeometryShape=Sphere  RectangleSize=[1 1]  RectangleSizeUnits=m  BrickDimensions=[1 1 1]  BrickDimensionUnits=m  CylinderRadius=1  CylinderRadiusUnits=m  CylinderLength=1  CylinderLengthUnits=m  SphereRadius=Earth.R  SphereRadiusUnits=m  EllipsoidRadii=[1 1 1]  EllipsoidRadiiUnits=m  ExtrusionCrossSection=[1 1; -1 1; -1 -1; 1 -1]  ExtrusionCrossSectionUnits=m  ExtrusionLength=1  ExtrusionLengthUnits=m  PolygonNumSides=3  PolygonOuterRadius=1  PolygonOuterRadiusUnits=m  ExtGeomFileType=STL  ExtGeomFileUnits=m  RevolutionCrossSection=[1 1; 1 -1; 2 -1; 2 1]  RevolutionCrossSectionUnits=m  RevolutionExtent=Full  RevolutionAngle=180  RevolutionAngleUnits=deg
  Earth Gravity : sm_lib/Forces and Torques/Gravitational Field  Mass=Earth.M  MassUnits=kg
      settings: SourceProductName=Simscape Multibody  SourceProductBaseCode=MS
  Conn1 : PMIOPort  Port=1  Side=Left
  connections:
  Conn1/RConn1 -- Earth/RConn1 -- Earth Gravity/LConn1

== matlab function Orbits/Reference ==
  data: t input; r1 output; r2 output; r3 output; orb_time input
function [r1,r2,r3] = fcn(t, orb_time)

%Define references r1 r2 r3 as a function of time. 

%Steps of amplitude A1 A2 A2 (deg) , at times T1 T2 T3 (sec)

T1 = 1*orb_time;
T2 = 2*orb_time;
T3 = 3*orb_time; 
A1 = 0.5 * (180/pi);
A2 = 0.5 * (180/pi);
A3 = 0.5 * (180/pi);

r1 = 0; r2 = 0; r3 = 0;

if t > T1; r1 = A1; end
if t > T2; r2 = A2; end
if t > T3; r3 = A3; end

return;

== matlab function Orbits/Dynamics/angleVectorPlane ==
  data: u input; delta output; a input; b input
function delta = angleVectorPlane(u,a,b)
%Tells the angle between a vector u = [u1, u2, u3], and a plane devined by
%the (non-parallel) vectors a and b

%Compute the normal vector N
N = cross(a,b);

delta = asin(abs(dot(N,u))/(norm(N)*norm(u))) ;

return;

== matlab function Orbits/Dynamics/ECEF2OrbitMatrix ==
  data: mu input; R_E_O output; l input; delta input
function R_E_O = ECEF2OrbitMatrix(mu,l,delta)
%Taking altitude mu, longitude l, and delta, angle between the
%velocity of le satellite and the (z_e, z_o) plane, gives the rotation
%matrix from ECEF to Orbit frame

%__________________________________________________________________________

cl = cos(l);
sl = sin(l);
cmu = cos(mu);
smu = sin(mu);
cd = cos(delta);
sd = sin(delta);


R_E_O = [-cl*smu*cd-sl*sd, cl*sd-sl*smu*cd, cmu*cd;
         cl*smu*sd-sl*cd, cl*cd + sl*smu*sd, -cl*cmu;
         -cl*cmu, -sl*cmu, -smu];
     
%R_E_O = R_E_O';

return;
